simulink model "Copy_of_TenMutantsTemplate"  (R2017b)
settings: Solver=ode3  StartTime=0.0  StopTime=inf  FixedStep=ts  RelTol=0.01  EnableMultiTasking=on
InitFcn:
  | ts=0.0005
  | %ts=100e-6;
StartFcn:
  | close all
StopFcn:
  | % Speed Torque Characterstic
  | 
  | 
  | %figure('Units','pixels', ...
  | %'Color',[1 1 1], ...
  | %'Name','Speed Torque Characterstic',...
  | %'NumberTitle','off',...
  | %'Position',[400 50 470 300], ...
  | %'ToolBar','none');
  | 
  | 
  | 
  | %plot(N_pi,Te_pi)
  | %title('Speed Torque Characterstic')
  | %xlabel('Speed [ RPM ]')
  | %ylabel('Electromagnetic Te_pi [ Nm ] ')
  | %grid on
  | %clear p4 p7 param5 param6 param8 parametres visible voltage
  | 
  | 
  | %clc
values from neighbouring files (symbols this model uses):
  TestOrder = [i]    [ExecuteTestSuite.m]    (also in mutants.m)
undefined symbols (not defined in the file or in its folder): emergency_button2, emergency_buttons, tc_simul, tc_size, temperature, trans1, trans2, trans3, trans4
libraries: simulink x44, powerlib_extras x11
(part 3 of 5)

== system Copy_of_TenMutantsTemplate/mutant7/PI Control1 ==
  N* : Inport
  N : Inport  Port=2
  Abs : Abs  SaturateOnIntegerOverflow=on
  Abs1 : Abs  SaturateOnIntegerOverflow=on
  Abs2 : Abs
  Compare To Constant : simulink/Logic and Bit Operations/Compare To Constant  relop=<=  const=0.1  OutDataTypeStr=uint8
  Constant : Constant  Value=0
  Divide : Product  Inputs=/*
  Integrator Limited : Integrator  LimitOutput=on  UpperSaturationLimit=30  LowerSaturationLimit=-30
  Proportional gain : Gain  Gain=0.8  SaturateOnIntegerOverflow=on  OutDataTypeStr=Inherit: Same as input  ParamDataTypeStr=Inherit: Same as input
  Rate Transition3 : RateTransition  OutPortSampleTimeOpt=Inherit
  Saturation : Saturate  UpperLimit=inf  LowerLimit=2
  Saturation2 : Saturate  UpperLimit=120  LowerLimit=0.02
  Sum1 : Sum  Inputs=|+-  SaturateOnIntegerOverflow=on  InputSameDT=on  OutDataTypeStr=Inherit: Same as first input
  Sum2 : Sum  SaturateOnIntegerOverflow=on  InputSameDT=on  OutDataTypeStr=Inherit: Same as first input
  Sum3 : Sum  Inputs=|++  SaturateOnIntegerOverflow=on  InputSameDT=on  OutDataTypeStr=Inherit: Same as first input
  Switch : Switch  Threshold=0.5
  ctrl_sat : Saturate  UpperLimit=30  LowerLimit=-30
  rpm2hz : Gain  Gain=4/120  SaturateOnIntegerOverflow=on  OutDataTypeStr=Inherit: Same as input  ParamDataTypeStr=Inherit: Same as input
  "rpm2hz  " : Gain  Gain=4/120  SaturateOnIntegerOverflow=on  OutDataTypeStr=Inherit: Same as input  ParamDataTypeStr=Inherit: Same as input
  Freq* : Outport
  wires:
  Saturation/1 -> Divide/1
  Switch/1 -> Integrator Limited/1
  Constant/1 -> Switch/3
  Compare To Constant/1 -> Switch/2
  Abs2/1 -> Divide/2
  Divide/1 -> Compare To Constant/1
  Integrator Limited/1 -> Sum2/1
  N/1 -> "rpm2hz  "/1
  Abs1/1 -> Sum1/2, Sum3/2
  Rate Transition3/1 -> Freq*/1
  Abs/1 -> Sum1/1, Saturation/1
  Sum1/1 -> Abs2/1, Switch/1, Proportional gain/1
  Saturation2/1 -> Rate Transition3/1
  "rpm2hz  "/1 -> Abs1/1
  Proportional gain/1 -> Sum2/2
  rpm2hz/1 -> Abs/1
  ctrl_sat/1 -> Sum3/1
  Sum3/1 -> Saturation2/1
  Sum2/1 -> ctrl_sat/1
  N*/1 -> rpm2hz/1

== system Copy_of_TenMutantsTemplate/mutant7/Subsystem ==
  Speed : Inport
  EmergButton1 : Inport  Port=2
  EmergButton2 : Inport  Port=3
  Temperature : Inport  Port=4
  Compare To Constant : simulink/Logic and Bit Operations/Compare To Constant  relop=>  const=100  OutDataTypeStr=boolean
  Compare To Constant1 : simulink/Logic and Bit Operations/Compare To Constant  relop===  const=0  OutDataTypeStr=boolean
  Constant : Constant  Value=emergency_buttons
  Constant1 : Constant  Value=temperature
  Constant2 : Constant  Value=emergency_button2
  Ir_a3 : Scope
  Logical Operator : Logic  Operator=OR  AllPortsSameDT=off  OutDataTypeStr=boolean
  Logical Operator1 : Logic  AllPortsSameDT=off  OutDataTypeStr=boolean
  Logical Operator2 : Logic  AllPortsSameDT=off  OutDataTypeStr=boolean
  Logical Operator3 : Logic  AllPortsSameDT=off  OutDataTypeStr=boolean
  Speed_to_0 : Constant  Value=0
  Switch : Switch  Criteria=u2 ~= 0
  Switch1 : Switch  Criteria=u2 ~= 0
  Switch2 : Switch  Criteria=u2 ~= 0
  Transfer Fcn1 : TransferFcn  Denominator=[20 1]
  "MotorSpeed " : Outport
  wires:
  EmergButton1/1 -> Logical Operator/1
  EmergButton2/1 -> Logical Operator3/1
  Logical Operator/1 -> Logical Operator1/1
  Speed/1 -> Transfer Fcn1/1
  Switch/1 -> Switch1/3
  Speed_to_0/1 -> Switch1/1, Switch/1
  Logical Operator1/1 -> Switch/2
  Constant/1 -> Logical Operator1/2
  Temperature/1 -> Compare To Constant/1
  Compare To Constant/1 -> Logical Operator2/1
  Constant1/1 -> Logical Operator2/2
  Logical Operator2/1 -> Switch1/2
  Logical Operator3/1 -> Logical Operator/2
  Constant2/1 -> Logical Operator3/2
  Switch1/1 -> Switch2/3, Switch2/1, Compare To Constant1/1
  Switch2/1 -> Ir_a3/1, "MotorSpeed "/1
  Compare To Constant1/1 -> Switch2/2
  Transfer Fcn1/1 -> Switch/3

== system Copy_of_TenMutantsTemplate/mutant7/VSI ==
  Freq : Inport
  Fcn : Fcn  Expr=(2*sqrt(2/3)*Vdc/3)*(2*u(1)-u(2)-u(3))
  Fcn1 : Fcn  Expr=(2*sqrt(2/3)*Vdc/3)*(2*u(2)-u(3)-u(1))
  Fcn2 : Fcn  Expr=(2*sqrt(2/3)*Vdc/3)*(2*u(3)-u(2)-u(1))
  SPWM : Subsystem
  Va : Outport
  Vb : Outport  Port=2
  Vc : Outport  Port=3
  wires:
  SPWM/1(g) -> Fcn2/1, Fcn/1, Fcn1/1
  Fcn1/1 -> Vb/1
  Fcn2/1 -> Vc/1
  Fcn/1 -> Va/1
  Freq/1 -> SPWM/1(Freq)

== system Copy_of_TenMutantsTemplate/mutant8/1 HP , 220 V Induction Motor ==
  tau : Inport
  V_a : Inport  Port=2
  V_b : Inport  Port=3
  V_c : Inport  Port=4
  Flux : Subsystem
  Measurements : Subsystem
  Mechanical : Subsystem
  Mux : Mux  Inputs=3
  Mux1 : Mux  Inputs=3
  abc to dq : Subsystem
  d_block : Subsystem
  dq to abc : Subsystem
  "dq to abc " : Subsystem
  q_block : Subsystem
  rad2rpm : Gain  Gain=30/pi
  m : Outport
  wires:
  Measurements/1(m) -> m/1
  rad2rpm/1 -> Measurements/8(N)
  Mux1/1 -> Measurements/2(I_r)
  Mux/1 -> Measurements/1(I_s)
  "dq to abc "/2(i_rb) -> Mux1/2
  "dq to abc "/3(i_rc) -> Mux1/3
  dq to abc/3(i_sc) -> Mux/3
  dq to abc/2(i_sb) -> Mux/2
  "dq to abc "/1(i_ra) -> Mux1/1
  dq to abc/1(i_sa) -> Mux/1
  V_a/1 -> abc to dq/1(Va)
  V_b/1 -> abc to dq/2(Vb)
  V_c/1 -> abc to dq/3(Vc)
  abc to dq/2(V_qs) -> Flux/2(V_qs)
  abc to dq/1(V_ds) -> Flux/1(V_ds)
  Flux/3(shi_qs) -> Mechanical/2(shi_qs), q_block/1(shi_qs)
  Flux/2("shi_dr ") -> d_block/2(shi_dr)
  tau/1 -> Mechanical/5(tau)
  Mechanical/1(Te) -> Measurements/7(Te)
  q_block/1(i_qs) -> Flux/5(I_qs), dq to abc/2(I_q), Measurements/5(I_qs), Measurements/4(I_dr), Mechanical/4(i_qs)
  q_block/2(i_qr) -> Flux/6(I_qr), "dq to abc "/2(I_q), Measurements/6(I_qr)
  d_block/2(i_dr) -> "dq to abc "/1(I_d), Flux/4(I_dr)
  d_block/1(i_ds) -> Flux/3(I_ds), dq to abc/1(I_d), Measurements/3(I_ds), Mechanical/3(i_ds)
  Flux/4("shi_qr ") -> q_block/2(shi_qr)
  Flux/1(shi_ds) -> Mechanical/1(shi_ds), d_block/1(shi_ds)
  Mechanical/3(we) -> Flux/7(we)
  Mechanical/2(omegaR) -> rad2rpm/1

== system Copy_of_TenMutantsTemplate/mutant8/Data Acquision ==
  note: DONE TO HAVE AN ALLOWABLE SIMULATION TIME
  m : Inport
  speed : Inport  Port=2
  2nd-Order Filter : powerlib_extras/Control  Blocks/2nd-Order Filter  FilterType=Lowpass  Fo=120  Zeta=0.707  Initialize=off  Vac_Init=[1 45 60]  Vdc_Init=-0.5  PlotResponse=off  param1=[1 500 1]
  Bus Selector : BusSelector  OutputSignals=Mechanical.Rotor Speed in (rpm),Mechanical.Electromagnetic Torque (N*m),Stator Measurement.Stator Current i_sa (A)
  Mux : Mux  Inputs=2
  filtroPasaBajos : TransferFcn  Denominator=[1 1]
  is_a : Outport
  Te(Nm) : Outport  Port=2
  wm : Outport  Port=3
  wm1 : Outport  Port=4
  wires:
  filtroPasaBajos/1 -> Mux/1, wm1/1
  Mux/1 -> wm/1
  speed/1 -> Mux/2
  Bus Selector/3 -> is_a/1  "<Stator Current i_sa (A)>"
  Bus Selector/1 -> filtroPasaBajos/1  "<Rotor Speed in (rpm)>"
  m/1 -> Bus Selector/1
  Bus Selector/2 -> 2nd-Order Filter/1  "<Electromagnetic Torque (N*m)>"
  2nd-Order Filter/1 -> Te(Nm)/1

== system Copy_of_TenMutantsTemplate/mutant8/PI Control1 ==
  N* : Inport
  N : Inport  Port=2
  Abs : Abs  SaturateOnIntegerOverflow=on
  Abs1 : Abs  SaturateOnIntegerOverflow=on
  Abs2 : Abs
  Compare To Constant : simulink/Logic and Bit Operations/Compare To Constant  relop=<=  const=0.1  OutDataTypeStr=uint8
  Constant : Constant  Value=0
  Divide : Product  Inputs=/*
  Integrator Limited : Integrator  LimitOutput=on  UpperSaturationLimit=30  LowerSaturationLimit=-30
  Proportional gain : Gain  Gain=0.8  SaturateOnIntegerOverflow=on  OutDataTypeStr=Inherit: Same as input  ParamDataTypeStr=Inherit: Same as input
  Rate Transition3 : RateTransition  OutPortSampleTimeOpt=Inherit
  Saturation : Saturate  UpperLimit=inf  LowerLimit=2
  Saturation2 : Saturate  UpperLimit=120  LowerLimit=0.02
  Sum1 : Sum  Inputs=|+-  SaturateOnIntegerOverflow=on  InputSameDT=on  OutDataTypeStr=Inherit: Same as first input
  Sum2 : Sum  SaturateOnIntegerOverflow=on  InputSameDT=on  OutDataTypeStr=Inherit: Same as first input
  Sum3 : Sum  Inputs=|++  SaturateOnIntegerOverflow=on  InputSameDT=on  OutDataTypeStr=Inherit: Same as first input
  Switch : Switch  Threshold=0.5
  ctrl_sat : Saturate  UpperLimit=30  LowerLimit=-30
  rpm2hz : Gain  Gain=4/120  SaturateOnIntegerOverflow=on  OutDataTypeStr=Inherit: Same as input  ParamDataTypeStr=Inherit: Same as input
  "rpm2hz  " : Gain  Gain=4/120  SaturateOnIntegerOverflow=on  OutDataTypeStr=Inherit: Same as input  ParamDataTypeStr=Inherit: Same as input
  Freq* : Outport
  wires:
  N*/1 -> rpm2hz/1
  Sum2/1 -> ctrl_sat/1
  Sum3/1 -> Saturation2/1
  ctrl_sat/1 -> Sum3/1
  rpm2hz/1 -> Abs/1
  Proportional gain/1 -> Sum2/2
  "rpm2hz  "/1 -> Abs1/1
  Saturation2/1 -> Rate Transition3/1
  Sum1/1 -> Proportional gain/1, Switch/1, Abs2/1
  Abs/1 -> Saturation/1, Sum1/1
  Rate Transition3/1 -> Freq*/1
  Abs1/1 -> Sum3/2, Sum1/2
  N/1 -> "rpm2hz  "/1
  Integrator Limited/1 -> Sum2/1
  Divide/1 -> Compare To Constant/1
  Abs2/1 -> Divide/2
  Compare To Constant/1 -> Switch/2
  Constant/1 -> Switch/3
  Switch/1 -> Integrator Limited/1
  Saturation/1 -> Divide/1

== system Copy_of_TenMutantsTemplate/mutant8/Subsystem ==
  Speed : Inport
  EmergButton1 : Inport  Port=2
  EmergButton2 : Inport  Port=3
  Temperature : Inport  Port=4
  Compare To Constant : simulink/Logic and Bit Operations/Compare To Constant  relop=>  const=100  OutDataTypeStr=boolean
  Compare To Constant1 : simulink/Logic and Bit Operations/Compare To Constant  relop===  const=0  OutDataTypeStr=boolean
  Constant : Constant  Value=emergency_buttons
  Constant1 : Constant  Value=temperature
  Constant2 : Constant  Value=emergency_button2
  Ir_a3 : Scope
  Logical Operator : Logic  Operator=OR  AllPortsSameDT=off  OutDataTypeStr=boolean
  Logical Operator1 : Logic  AllPortsSameDT=off  OutDataTypeStr=boolean
  Logical Operator2 : Logic  AllPortsSameDT=off  OutDataTypeStr=boolean
  Logical Operator3 : Logic  AllPortsSameDT=off  OutDataTypeStr=boolean
  Speed_to_0 : Constant  Value=0
  Switch : Switch  Criteria=u2 ~= 0
  Switch1 : Switch  Criteria=u2 ~= 0
  Switch2 : Switch  Criteria=u2 ~= 0
  Transfer Fcn1 : TransferFcn  Denominator=[20 1]
  "MotorSpeed " : Outport
  wires:
  Transfer Fcn1/1 -> Switch/3
  Compare To Constant1/1 -> Switch2/2
  Switch2/1 -> "MotorSpeed "/1, Ir_a3/1
  Switch1/1 -> Compare To Constant1/1, Switch2/1, Switch2/3
  Constant2/1 -> Logical Operator3/2
  Logical Operator3/1 -> Logical Operator/2
  Logical Operator2/1 -> Switch1/2
  Constant1/1 -> Logical Operator2/2
  Compare To Constant/1 -> Logical Operator2/1
  Temperature/1 -> Compare To Constant/1
  Constant/1 -> Logical Operator1/2
  Logical Operator1/1 -> Switch/2
  Speed_to_0/1 -> Switch/1, Switch1/1
  Switch/1 -> Switch1/3
  Speed/1 -> Transfer Fcn1/1
  Logical Operator/1 -> Logical Operator1/1
  EmergButton2/1 -> Logical Operator3/1
  EmergButton1/1 -> Logical Operator/1

== system Copy_of_TenMutantsTemplate/mutant8/VSI ==
  Freq : Inport
  Fcn : Fcn  Expr=(2*sqrt(2/3)*Vdc/3)*(2*u(1)-u(2)-u(3))
  Fcn1 : Fcn  Expr=(2*sqrt(2/3)*Vdc/3)*(2*u(2)-u(3)-u(1))
  Fcn2 : Fcn  Expr=(2*sqrt(2/3)*Vdc/3)*(2*u(3)-u(2)-u(1))
  SPWM : Subsystem
  Va : Outport
  Vb : Outport  Port=2
  Vc : Outport  Port=3
  wires:
  Freq/1 -> SPWM/1(Freq)
  Fcn/1 -> Va/1
  Fcn2/1 -> Vc/1
  Fcn1/1 -> Vb/1
  SPWM/1(g) -> Fcn1/1, Fcn/1, Fcn2/1

== system Copy_of_TenMutantsTemplate/mutant9/1 HP , 220 V Induction Motor ==
  tau : Inport
  V_a : Inport  Port=2
  V_b : Inport  Port=3
  V_c : Inport  Port=4
  Flux : Subsystem
  Measurements : Subsystem
  Mechanical : Subsystem
  Mux : Mux  Inputs=3
  Mux1 : Mux  Inputs=3
  abc to dq : Subsystem
  d_block : Subsystem
  dq to abc : Subsystem
  "dq to abc " : Subsystem
  q_block : Subsystem
  rad2rpm : Gain  Gain=30/pi
  m : Outport
  wires:
  Mechanical/2(omegaR) -> rad2rpm/1
  Mechanical/3(we) -> Flux/7(we)
  Flux/1(shi_ds) -> d_block/1(shi_ds), Mechanical/1(shi_ds)
  Flux/4("shi_qr ") -> q_block/2(shi_qr)
  d_block/1(i_ds) -> Mechanical/3(i_ds), Measurements/3(I_ds), dq to abc/1(I_d), Flux/3(I_ds)
  d_block/2(i_dr) -> Flux/4(I_dr), "dq to abc "/1(I_d)
  q_block/2(i_qr) -> Measurements/6(I_qr), "dq to abc "/2(I_q), Flux/6(I_qr)
  q_block/1(i_qs) -> Mechanical/4(i_qs), Measurements/4(I_dr), Measurements/5(I_qs), dq to abc/2(I_q), Flux/5(I_qs)
  Mechanical/1(Te) -> Measurements/7(Te)
  tau/1 -> Mechanical/5(tau)
  Flux/2("shi_dr ") -> d_block/2(shi_dr)
  Flux/3(shi_qs) -> q_block/1(shi_qs), Mechanical/2(shi_qs)
  abc to dq/1(V_ds) -> Flux/1(V_ds)
  abc to dq/2(V_qs) -> Flux/2(V_qs)
  V_c/1 -> abc to dq/3(Vc)
  V_b/1 -> abc to dq/2(Vb)
  V_a/1 -> abc to dq/1(Va)
  dq to abc/1(i_sa) -> Mux/1
  "dq to abc "/1(i_ra) -> Mux1/1
  dq to abc/2(i_sb) -> Mux/2
  dq to abc/3(i_sc) -> Mux/3
  "dq to abc "/3(i_rc) -> Mux1/3
  "dq to abc "/2(i_rb) -> Mux1/2
  Mux/1 -> Measurements/1(I_s)
  Mux1/1 -> Measurements/2(I_r)
  rad2rpm/1 -> Measurements/8(N)
  Measurements/1(m) -> m/1

== system Copy_of_TenMutantsTemplate/mutant9/Data Acquision ==
  note: DONE TO HAVE AN ALLOWABLE SIMULATION TIME
  m : Inport
  speed : Inport  Port=2
  2nd-Order Filter : powerlib_extras/Control  Blocks/2nd-Order Filter  FilterType=Lowpass  Fo=120  Zeta=0.707  Initialize=off  Vac_Init=[1 45 60]  Vdc_Init=-0.5  PlotResponse=off  param1=[1 500 1]
  Bus Selector : BusSelector  OutputSignals=Mechanical.Rotor Speed in (rpm),Mechanical.Electromagnetic Torque (N*m),Stator Measurement.Stator Current i_sa (A)
  Mux : Mux  Inputs=2
  filtroPasaBajos : TransferFcn  Denominator=[1 1]
  is_a : Outport
  Te(Nm) : Outport  Port=2
  wm : Outport  Port=3
  wm1 : Outport  Port=4
  wires:
  2nd-Order Filter/1 -> Te(Nm)/1
  Bus Selector/2 -> 2nd-Order Filter/1  "<Electromagnetic Torque (N*m)>"
  m/1 -> Bus Selector/1
  Bus Selector/1 -> filtroPasaBajos/1  "<Rotor Speed in (rpm)>"
  Bus Selector/3 -> is_a/1  "<Stator Current i_sa (A)>"
  speed/1 -> Mux/2
  Mux/1 -> wm/1
  filtroPasaBajos/1 -> wm1/1, Mux/1

== system Copy_of_TenMutantsTemplate/mutant9/PI Control1 ==
  N* : Inport
  N : Inport  Port=2
  Abs : Abs  SaturateOnIntegerOverflow=on
  Abs1 : Abs  SaturateOnIntegerOverflow=on
  Abs2 : Abs
  Compare To Constant : simulink/Logic and Bit Operations/Compare To Constant  relop=<=  const=0.1  OutDataTypeStr=uint8
  Constant : Constant  Value=0
  Divide : Product  Inputs=/*
  Integrator Limited : Integrator  LimitOutput=on  UpperSaturationLimit=30  LowerSaturationLimit=-30
  Proportional gain : Gain  Gain=0.8  SaturateOnIntegerOverflow=on  OutDataTypeStr=Inherit: Same as input  ParamDataTypeStr=Inherit: Same as input
  Rate Transition3 : RateTransition  OutPortSampleTimeOpt=Inherit
  Saturation : Saturate  UpperLimit=inf  LowerLimit=2
  Saturation2 : Saturate  UpperLimit=120  LowerLimit=0.02
  Sum1 : Sum  Inputs=|+-  SaturateOnIntegerOverflow=on  InputSameDT=on  OutDataTypeStr=Inherit: Same as first input
  Sum2 : Sum  SaturateOnIntegerOverflow=on  InputSameDT=on  OutDataTypeStr=Inherit: Same as first input
  Sum3 : Sum  Inputs=|++  SaturateOnIntegerOverflow=on  InputSameDT=on  OutDataTypeStr=Inherit: Same as first input
  Switch : Switch  Threshold=0.5
  ctrl_sat : Saturate  UpperLimit=30  LowerLimit=-30
  rpm2hz : Gain  Gain=4/120  SaturateOnIntegerOverflow=on  OutDataTypeStr=Inherit: Same as input  ParamDataTypeStr=Inherit: Same as input
  "rpm2hz  " : Gain  Gain=4/120  SaturateOnIntegerOverflow=on  OutDataTypeStr=Inherit: Same as input  ParamDataTypeStr=Inherit: Same as input
  Freq* : Outport
  wires:
  Saturation/1 -> Divide/1
  Switch/1 -> Integrator Limited/1
  Constant/1 -> Switch/3
  Compare To Constant/1 -> Switch/2
  Abs2/1 -> Divide/2
  Divide/1 -> Compare To Constant/1
  Integrator Limited/1 -> Sum2/1
  N/1 -> "rpm2hz  "/1
  Abs1/1 -> Sum1/2, Sum3/2
  Rate Transition3/1 -> Freq*/1
  Abs/1 -> Sum1/1, Saturation/1
  Sum1/1 -> Abs2/1, Switch/1, Proportional gain/1
  Saturation2/1 -> Rate Transition3/1
  "rpm2hz  "/1 -> Abs1/1
  Proportional gain/1 -> Sum2/2
  rpm2hz/1 -> Abs/1
  ctrl_sat/1 -> Sum3/1
  Sum3/1 -> Saturation2/1
  Sum2/1 -> ctrl_sat/1
  N*/1 -> rpm2hz/1

== system Copy_of_TenMutantsTemplate/mutant9/Subsystem ==
  Speed : Inport
  EmergButton1 : Inport  Port=2
  EmergButton2 : Inport  Port=3
  Temperature : Inport  Port=4
  Compare To Constant : simulink/Logic and Bit Operations/Compare To Constant  relop=>  const=100  OutDataTypeStr=boolean
  Compare To Constant1 : simulink/Logic and Bit Operations/Compare To Constant  relop===  const=0  OutDataTypeStr=boolean
  Constant : Constant  Value=emergency_buttons
  Constant1 : Constant  Value=temperature
  Constant2 : Constant  Value=emergency_button2
  Ir_a3 : Scope
  Logical Operator : Logic  Operator=OR  AllPortsSameDT=off  OutDataTypeStr=boolean
  Logical Operator1 : Logic  AllPortsSameDT=off  OutDataTypeStr=boolean
  Logical Operator2 : Logic  AllPortsSameDT=off  OutDataTypeStr=boolean
  Logical Operator3 : Logic  AllPortsSameDT=off  OutDataTypeStr=boolean
  Speed_to_0 : Constant  Value=0
  Switch : Switch  Criteria=u2 ~= 0
  Switch1 : Switch  Criteria=u2 ~= 0
  Switch2 : Switch  Criteria=u2 ~= 0
  Transfer Fcn1 : TransferFcn  Denominator=[20 1]
  "MotorSpeed " : Outport
  wires:
  EmergButton1/1 -> Logical Operator/1
  EmergButton2/1 -> Logical Operator3/1
  Logical Operator/1 -> Logical Operator1/1
  Speed/1 -> Transfer Fcn1/1
  Switch/1 -> Switch1/3
  Speed_to_0/1 -> Switch1/1, Switch/1
  Logical Operator1/1 -> Switch/2
  Constant/1 -> Logical Operator1/2
  Temperature/1 -> Compare To Constant/1
  Compare To Constant/1 -> Logical Operator2/1
  Constant1/1 -> Logical Operator2/2
  Logical Operator2/1 -> Switch1/2
  Logical Operator3/1 -> Logical Operator/2
  Constant2/1 -> Logical Operator3/2
  Switch1/1 -> Switch2/3, Switch2/1, Compare To Constant1/1
  Switch2/1 -> Ir_a3/1, "MotorSpeed "/1
  Compare To Constant1/1 -> Switch2/2
  Transfer Fcn1/1 -> Switch/3

== system Copy_of_TenMutantsTemplate/mutant9/VSI ==
  Freq : Inport
  Fcn : Fcn  Expr=(2*sqrt(2/3)*Vdc/3)*(2*u(1)-u(2)-u(3))
  Fcn1 : Fcn  Expr=(2*sqrt(2/3)*Vdc/3)*(2*u(2)-u(3)-u(1))
  Fcn2 : Fcn  Expr=(2*sqrt(2/3)*Vdc/3)*(2*u(3)-u(2)-u(1))
  SPWM : Subsystem
  Va : Outport
  Vb : Outport  Port=2
  Vc : Outport  Port=3
  wires:
  SPWM/1(g) -> Fcn2/1, Fcn/1, Fcn1/1
  Fcn1/1 -> Vb/1
  Fcn2/1 -> Vc/1
  Fcn/1 -> Va/1
  Freq/1 -> SPWM/1(Freq)

== system Copy_of_TenMutantsTemplate/System/1 HP , 220 V Induction Motor/Flux ==
  V_ds : Inport
  V_qs : Inport  Port=2
  I_ds : Inport  Port=3
  I_dr : Inport  Port=4
  I_qs : Inport  Port=5
  I_qr : Inport  Port=6
  we : Inport  Port=7
  Integrator{,1..3} (4 alike) : Integrator
  Product : Product
  Product1 : Product
  Rr : Gain  Gain=Rr
  "Rr " : Gain  Gain=Rr
  Rs : Gain  Gain=Rs
  "Rs " : Gain  Gain=Rs
  Sum : Sum  Inputs=+|-
  Sum1 : Sum  Inputs=+|-
  Sum2 : Sum  Inputs=|--
  Sum3 : Sum  Inputs=|+-
  shi_ds : Outport
  "shi_dr " : Outport  Port=2
  shi_qs : Outport  Port=3
  "shi_qr " : Outport  Port=4
  wires:
  Sum3/1 -> Integrator3/1
  "Rr "/1 -> Sum3/2
  Product1/1 -> Sum3/1
  I_qr/1 -> "Rr "/1
  Integrator2/1 -> "shi_dr "/1, Product1/2
  Sum2/1 -> Integrator2/1
  Product/1 -> Sum2/1
  Rr/1 -> Sum2/2
  I_dr/1 -> Rr/1
  Integrator3/1 -> "shi_qr "/1, Product/1
  we/1 -> Product1/1, Product/2
  "Rs "/1 -> Sum1/2
  Rs/1 -> Sum/2
  Integrator1/1 -> shi_qs/1
  Integrator/1 -> shi_ds/1
  Sum1/1 -> Integrator1/1
  V_qs/1 -> Sum1/1
  I_qs/1 -> "Rs "/1
  Sum/1 -> Integrator/1
  V_ds/1 -> Sum/1
  I_ds/1 -> Rs/1

== system Copy_of_TenMutantsTemplate/System/1 HP , 220 V Induction Motor/Measurements ==
  I_s : Inport
  I_r : Inport  Port=2
  I_ds : Inport  Port=3
  I_dr : Inport  Port=4
  I_qs : Inport  Port=5
  I_qr : Inport  Port=6
  Te : Inport  Port=7
  N : Inport  Port=8
  Bus Creator : BusCreator  Inputs=5
  Bus Creator1 : BusCreator  Inputs=5
  Bus Creator2 : BusCreator  Inputs=2
  Bus Creator3 : BusCreator  Inputs=3
  Demux : Demux  Outputs=3
  Demux1 : Demux  Outputs=3
  m : Outport
  wires:
  Bus Creator3/1 -> m/1
  Bus Creator2/1 -> Bus Creator3/3  "Mechanical"
  Bus Creator1/1 -> Bus Creator3/2  "Rotor Measurement"
  Bus Creator/1 -> Bus Creator3/1  "Stator Measurement"
  N/1 -> Bus Creator2/2  "Rotor Speed in (rpm)"
  Te/1 -> Bus Creator2/1  "Electromagnetic Torque (N*m)"
  I_qr/1 -> Bus Creator1/5  "Rotor Current i_qs (A)"
  I_dr/1 -> Bus Creator1/4  "Rotor Current i_ds (A)"
  Demux1/3 -> Bus Creator1/3  "Rotor Current i_sc (A)"
  Demux1/2 -> Bus Creator1/2  "Rotor Current i_sb (A)"
  Demux1/1 -> Bus Creator1/1  "Rotor Current i_sa (A)"
  I_r/1 -> Demux1/1
  I_qs/1 -> Bus Creator/5  "Stator Current i_qs (A)"
  I_ds/1 -> Bus Creator/4  "Stator Current i_ds (A)"
  Demux/3 -> Bus Creator/3  "Stator Current i_sc (A)"
  Demux/2 -> Bus Creator/2  "Stator Current i_sb (A)"
  Demux/1 -> Bus Creator/1  "Stator Current i_sa (A)"
  I_s/1 -> Demux/1

== system Copy_of_TenMutantsTemplate/System/1 HP , 220 V Induction Motor/Mechanical ==
  shi_ds : Inport
  shi_qs : Inport  Port=2
  i_ds : Inport  Port=3
  i_qs : Inport  Port=4
  tau : Inport  Port=5
  " " : Gain  Gain=P/2  SaturateOnIntegerOverflow=on  OutDataTypeStr=Inherit: Same as input  ParamDataTypeStr=Inherit: Same as input
  "  " : Gain  Gain=3*P/4  SaturateOnIntegerOverflow=on  OutDataTypeStr=Inherit: Same as input  ParamDataTypeStr=Inherit: Same as input
  1/J : Gain  Gain=1/J  SaturateOnIntegerOverflow=on  OutDataTypeStr=Inherit: Same as input  ParamDataTypeStr=Inherit: Same as input
  Integratorw : Integrator
  Product1 : Product
  Product2 : Product
  Sum : Sum  Inputs=+|-
  Sum5 : Sum  Inputs=+-  SaturateOnIntegerOverflow=on  InputSameDT=on  OutDataTypeStr=Inherit: Same as first input
  Te : Outport
  omegaR : Outport  Port=2
  we : Outport  Port=3
  wires:
  " "/1 -> we/1
  Integratorw/1 -> omegaR/1, " "/1
  1/J/1 -> Integratorw/1
  Sum5/1 -> 1/J/1
  tau/1 -> Sum5/2
  "  "/1 -> Sum5/1, Te/1
  Sum/1 -> "  "/1
  Product2/1 -> Sum/1
  Product1/1 -> Sum/2
  i_ds/1 -> Product1/2
  shi_qs/1 -> Product1/1
  i_qs/1 -> Product2/2
  shi_ds/1 -> Product2/1

== system Copy_of_TenMutantsTemplate/System/1 HP , 220 V Induction Motor/abc to dq ==
  Va : Inport
  Vb : Inport  Port=2
  Vc : Inport  Port=3
  "            " : Terminator
  Demux : Demux  Outputs=3
  Mux : Mux  Inputs=3
  abc2dq : Gain  Gain=[2/3 -1/3 -1/3; 0 sqrt(3)/3 -sqrt(3)/3; 1/3 1/3 1/3]  Multiplication=Matrix(K*u)  SaturateOnIntegerOverflow=on  OutDataTypeStr=Inherit: Same as input  ParamDataTypeStr=Inherit: Same as input
  V_ds : Outport
  V_qs : Outport  Port=2
  wires:
  Mux/1 -> abc2dq/1
  abc2dq/1 -> Demux/1
  Demux/2 -> V_qs/1
  Demux/1 -> V_ds/1
  Va/1 -> Mux/1
  Vb/1 -> Mux/2
  Vc/1 -> Mux/3
  Demux/3 -> "            "/1

== system Copy_of_TenMutantsTemplate/System/1 HP , 220 V Induction Motor/d_block ==
  shi_ds : Inport
  shi_dr : Inport  Port=2
  1/(Lr-((Lm*Lm)/Ls)) : Gain  Gain=1/(Lr-((Lm*Lm)/Ls))  SaturateOnIntegerOverflow=on  OutDataTypeStr=Inherit: Same as input  ParamDataTypeStr=Inherit: Same as input
  1/(Ls-((Lm*Lm)/Lr)) : Gain  Gain=1/(Ls-((Lm*Lm)/Lr))  SaturateOnIntegerOverflow=on  OutDataTypeStr=Inherit: Same as input  ParamDataTypeStr=Inherit: Same as input
  Lm/Lr : Gain  Gain=Lm/Lr
  Lm/Ls : Gain  Gain=Lm/Ls
  Sum : Sum  Inputs=|+-
  Sum1 : Sum  Inputs=-+|
  i_ds : Outport
  i_dr : Outport  Port=2
  wires:
  Sum1/1 -> 1/(Lr-((Lm*Lm)/Ls))/1
  Lm/Ls/1 -> Sum1/1
  Sum/1 -> 1/(Ls-((Lm*Lm)/Lr))/1
  Lm/Lr/1 -> Sum/2
  shi_dr/1 -> Sum1/2, Lm/Lr/1
  shi_ds/1 -> Lm/Ls/1, Sum/1
  1/(Lr-((Lm*Lm)/Ls))/1 -> i_dr/1
  1/(Ls-((Lm*Lm)/Lr))/1 -> i_ds/1

== system Copy_of_TenMutantsTemplate/System/1 HP , 220 V Induction Motor/dq to abc ==
  I_d : Inport
  I_q : Inport  Port=2
  Demux : Demux  Outputs=3
  Gain : Gain  Gain=2/3  SaturateOnIntegerOverflow=on  OutDataTypeStr=Inherit: Same as input  ParamDataTypeStr=Inherit: Same as input
  Matrix Gain : Gain  Gain=[1 0;-0.5 -sqrt(3)/2;-0.5 sqrt(3)/2]  Multiplication=Matrix(K*u)  SaturateOnIntegerOverflow=on  OutDataTypeStr=Inherit: Same as input  ParamDataTypeStr=Inherit: Same as input
  Mux : Mux  Inputs=2
  i_sa : Outport
  i_sb : Outport  Port=2
  i_sc : Outport  Port=3
  wires:
  Demux/1 -> i_sa/1
  Demux/3 -> i_sc/1
  I_q/1 -> Mux/2
  I_d/1 -> Mux/1
  Demux/2 -> i_sb/1
  Matrix Gain/1 -> Gain/1
  Gain/1 -> Demux/1
  Mux/1 -> Matrix Gain/1

== system Copy_of_TenMutantsTemplate/System/1 HP , 220 V Induction Motor/dq to abc  ==
  I_d : Inport
  I_q : Inport  Port=2
  Demux : Demux  Outputs=3
  Gain : Gain  Gain=2/3  SaturateOnIntegerOverflow=on  OutDataTypeStr=Inherit: Same as input  ParamDataTypeStr=Inherit: Same as input
  Matrix Gain : Gain  Gain=[1 0;-0.5 -sqrt(3)/2;-0.5 sqrt(3)/2]  Multiplication=Matrix(K*u)  SaturateOnIntegerOverflow=on  OutDataTypeStr=Inherit: Same as input  ParamDataTypeStr=Inherit: Same as input
  Mux : Mux  Inputs=2
  i_ra : Outport
  i_rb : Outport  Port=2
  i_rc : Outport  Port=3
  wires:
  Mux/1 -> Matrix Gain/1
  Gain/1 -> Demux/1
  Matrix Gain/1 -> Gain/1
  Demux/2 -> i_rb/1
  I_d/1 -> Mux/1
  I_q/1 -> Mux/2
  Demux/3 -> i_rc/1
  Demux/1 -> i_ra/1

== system Copy_of_TenMutantsTemplate/System/1 HP , 220 V Induction Motor/q_block ==
  shi_qs : Inport
  shi_qr : Inport  Port=2
  1/(Lr-((Lm*Lm)/Ls)) : Gain  Gain=1/(Lr-((Lm*Lm)/Ls))  SaturateOnIntegerOverflow=on  OutDataTypeStr=Inherit: Same as input  ParamDataTypeStr=Inherit: Same as input
  1/(Ls-((Lm*Lm)/Lr)) : Gain  Gain=1/(Ls-((Lm*Lm)/Lr))  SaturateOnIntegerOverflow=on  OutDataTypeStr=Inherit: Same as input  ParamDataTypeStr=Inherit: Same as input
  Lm/Lr : Gain  Gain=Lm/Lr
  Lm/Ls : Gain  Gain=Lm/Ls
  Sum : Sum  Inputs=|+-
  Sum1 : Sum  Inputs=-+|
  i_qs : Outport
  i_qr : Outport  Port=2
  wires:
  Sum1/1 -> 1/(Lr-((Lm*Lm)/Ls))/1
  Lm/Ls/1 -> Sum1/1
  Sum/1 -> 1/(Ls-((Lm*Lm)/Lr))/1
  Lm/Lr/1 -> Sum/2
  shi_qr/1 -> Lm/Lr/1, Sum1/2
  shi_qs/1 -> Lm/Ls/1, Sum/1
  1/(Lr-((Lm*Lm)/Ls))/1 -> i_qr/1
  1/(Ls-((Lm*Lm)/Lr))/1 -> i_qs/1

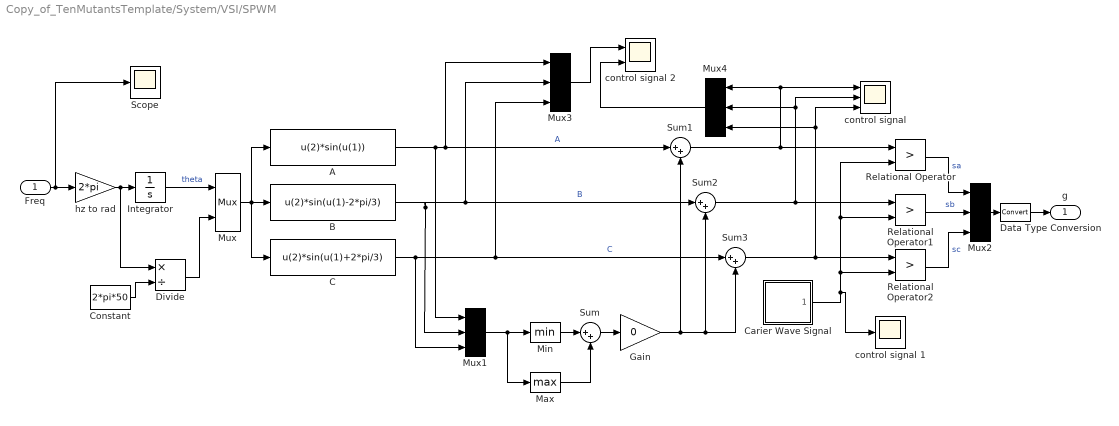
== system Copy_of_TenMutantsTemplate/System/VSI/SPWM ==
  Freq : Inport
  A : Fcn  Expr=u(2)*sin(u(1))
  B : Fcn  Expr=u(2)*sin(u(1)-2*pi/3)
  C : Fcn  Expr=u(2)*sin(u(1)+2*pi/3)
  Carier Wave Signal : Subsystem  mask(Carrier Wave Generator:){A=1, fc=500}
      mask prompts: A "Amplitude"; fc "Carrier Wave Frequency"
      mask Display: fprintf('Carrier\nWave')
  Constant : Constant  Value=2*pi*50
  Data Type Conversion : DataTypeConversion
  Divide : Product  Inputs=*/
  Gain : Gain  Gain=0
  Integrator : Integrator
  Max : MinMax  Function=max
  Min : MinMax
  Mux : Mux  Inputs=2
      settings: DisplayOption=signals
  Mux{1..4} (4 alike) : Mux  Inputs=3
      settings: DisplayOption=signals
  Relational Operator : RelationalOperator  Operator=>  OutDataTypeStr=boolean  RndMeth=Nearest
  Relational Operator1 : RelationalOperator  Operator=>  OutDataTypeStr=boolean  RndMeth=Nearest
  Relational Operator2 : RelationalOperator  Operator=>  OutDataTypeStr=boolean  RndMeth=Nearest
  Scope : Scope
  Sum{,1..3} (4 alike) : Sum  Inputs=|++
  "control signal " : Scope  NumInputPorts=3
  control signal 1 : Scope
  control signal 2 : Scope  NumInputPorts=2
  hz to rad : Gain  Gain=2*pi
  g : Outport
  wires:
  Mux4/1 -> control signal 2/2
  Mux3/1 -> control signal 2/1
  Constant/1 -> Divide/2
  Divide/1 -> Mux/2
  Gain/1 -> Sum1/2, Sum3/2, Sum2/2
  Freq/1 -> hz to rad/1, Scope/1
  C/1 -> Mux3/3, Sum3/1, Mux1/3  "C"
  Mux/1 -> C/1, A/1, B/1
  Integrator/1 -> Mux/1  "theta"
  A/1 -> Mux3/1, Sum1/1, Mux1/1  "A"
  hz to rad/1 -> Divide/1, Integrator/1
  B/1 -> Mux3/2, Sum2/1, Mux1/2  "B"
  Min/1 -> Sum/1
  Max/1 -> Sum/2
  Carier Wave Signal/1("Carier Wave ") -> control signal 1/1, Relational Operator2/2, Relational Operator1/2, Relational Operator/2
  Relational Operator2/1 -> Mux2/3  "sc"
  Relational Operator1/1 -> Mux2/2  "sb"
  Relational Operator/1 -> Mux2/1  "sa"
  Mux1/1 -> Max/1, Min/1
  Sum/1 -> Gain/1
  Sum1/1 -> Mux4/1, "control signal "/1, Relational Operator/1
  Sum2/1 -> Mux4/2, "control signal "/2, Relational Operator1/1
  Sum3/1 -> Mux4/3, "control signal "/3, Relational Operator2/1
  Mux2/1 -> Data Type Conversion/1
  Data Type Conversion/1 -> g/1

== system Copy_of_TenMutantsTemplate/mutant1/1 HP , 220 V Induction Motor/Flux ==
  V_ds : Inport
  V_qs : Inport  Port=2
  I_ds : Inport  Port=3
  I_dr : Inport  Port=4
  I_qs : Inport  Port=5
  I_qr : Inport  Port=6
  we : Inport  Port=7
  Integrator{,1..3} (4 alike) : Integrator
  Product : Product
  Product1 : Product
  Rr : Gain  Gain=Rr
  "Rr " : Gain  Gain=Rr
  Rs : Gain  Gain=Rs
  "Rs " : Gain  Gain=Rs
  Sum : Sum  Inputs=+|-
  Sum1 : Sum  Inputs=+|-
  Sum2 : Sum  Inputs=|--
  Sum3 : Sum  Inputs=|+-
  shi_ds : Outport
  "shi_dr " : Outport  Port=2
  shi_qs : Outport  Port=3
  "shi_qr " : Outport  Port=4
  wires:
  I_ds/1 -> Rs/1
  V_ds/1 -> Sum/1
  Sum/1 -> Integrator/1
  I_qs/1 -> "Rs "/1
  V_qs/1 -> Sum1/1
  Sum1/1 -> Integrator1/1
  Integrator/1 -> shi_ds/1
  Integrator1/1 -> shi_qs/1
  Rs/1 -> Sum/2
  "Rs "/1 -> Sum1/2
  we/1 -> Product/2, Product1/1
  Integrator3/1 -> Product/1, "shi_qr "/1
  I_dr/1 -> Rr/1
  Rr/1 -> Sum2/2
  Product/1 -> Sum2/1
  Sum2/1 -> Integrator2/1
  Integrator2/1 -> Product1/2, "shi_dr "/1
  I_qr/1 -> "Rr "/1
  Product1/1 -> Sum3/1
  "Rr "/1 -> Sum3/2
  Sum3/1 -> Integrator3/1

== system Copy_of_TenMutantsTemplate/mutant1/1 HP , 220 V Induction Motor/Measurements ==
  I_s : Inport
  I_r : Inport  Port=2
  I_ds : Inport  Port=3
  I_dr : Inport  Port=4
  I_qs : Inport  Port=5
  I_qr : Inport  Port=6
  Te : Inport  Port=7
  N : Inport  Port=8
  Bus Creator : BusCreator  Inputs=5
  Bus Creator1 : BusCreator  Inputs=5
  Bus Creator2 : BusCreator  Inputs=2
  Bus Creator3 : BusCreator  Inputs=3
  Demux : Demux  Outputs=3
  Demux1 : Demux  Outputs=3
  m : Outport
  wires:
  I_s/1 -> Demux/1
  Demux/1 -> Bus Creator/1  "Stator Current i_sa (A)"
  Demux/2 -> Bus Creator/2  "Stator Current i_sb (A)"
  Demux/3 -> Bus Creator/3  "Stator Current i_sc (A)"
  I_ds/1 -> Bus Creator/4  "Stator Current i_ds (A)"
  I_qs/1 -> Bus Creator/5  "Stator Current i_qs (A)"
  I_r/1 -> Demux1/1
  Demux1/1 -> Bus Creator1/1  "Rotor Current i_sa (A)"
  Demux1/2 -> Bus Creator1/2  "Rotor Current i_sb (A)"
  Demux1/3 -> Bus Creator1/3  "Rotor Current i_sc (A)"
  I_dr/1 -> Bus Creator1/4  "Rotor Current i_ds (A)"
  I_qr/1 -> Bus Creator1/5  "Rotor Current i_qs (A)"
  Te/1 -> Bus Creator2/1  "Electromagnetic Torque (N*m)"
  N/1 -> Bus Creator2/2  "Rotor Speed in (rpm)"
  Bus Creator/1 -> Bus Creator3/1  "Stator Measurement"
  Bus Creator1/1 -> Bus Creator3/2  "Rotor Measurement"
  Bus Creator2/1 -> Bus Creator3/3  "Mechanical"
  Bus Creator3/1 -> m/1

== system Copy_of_TenMutantsTemplate/mutant1/1 HP , 220 V Induction Motor/Mechanical ==
  shi_ds : Inport
  shi_qs : Inport  Port=2
  i_ds : Inport  Port=3
  i_qs : Inport  Port=4
  tau : Inport  Port=5
  " " : Gain  Gain=P/2  SaturateOnIntegerOverflow=on  OutDataTypeStr=Inherit: Same as input  ParamDataTypeStr=Inherit: Same as input
  "  " : Gain  Gain=3*P/4  SaturateOnIntegerOverflow=on  OutDataTypeStr=Inherit: Same as input  ParamDataTypeStr=Inherit: Same as input
  1/J : Gain  Gain=1/J  SaturateOnIntegerOverflow=on  OutDataTypeStr=Inherit: Same as input  ParamDataTypeStr=Inherit: Same as input
  Integratorw : Integrator
  Product1 : Product
  Product2 : Product
  Sum : Sum  Inputs=+|-
  Sum5 : Sum  Inputs=+-  SaturateOnIntegerOverflow=on  InputSameDT=on  OutDataTypeStr=Inherit: Same as first input
  Te : Outport
  omegaR : Outport  Port=2
  we : Outport  Port=3
  wires:
  shi_ds/1 -> Product2/1
  i_qs/1 -> Product2/2
  shi_qs/1 -> Product1/1
  i_ds/1 -> Product1/2
  Product1/1 -> Sum/2
  Product2/1 -> Sum/1
  Sum/1 -> "  "/1
  "  "/1 -> Te/1, Sum5/1
  tau/1 -> Sum5/2
  Sum5/1 -> 1/J/1
  1/J/1 -> Integratorw/1
  Integratorw/1 -> " "/1, omegaR/1
  " "/1 -> we/1

== system Copy_of_TenMutantsTemplate/mutant1/1 HP , 220 V Induction Motor/abc to dq ==
  Va : Inport
  Vb : Inport  Port=2
  Vc : Inport  Port=3
  "            " : Terminator
  Demux : Demux  Outputs=3
  Mux : Mux  Inputs=3
  abc2dq : Gain  Gain=[2/3 -1/3 -1/3; 0 sqrt(3)/3 -sqrt(3)/3; 1/3 1/3 1/3]  Multiplication=Matrix(K*u)  SaturateOnIntegerOverflow=on  OutDataTypeStr=Inherit: Same as input  ParamDataTypeStr=Inherit: Same as input
  V_ds : Outport
  V_qs : Outport  Port=2
  wires:
  Demux/3 -> "            "/1
  Vc/1 -> Mux/3
  Vb/1 -> Mux/2
  Va/1 -> Mux/1
  Demux/1 -> V_ds/1
  Demux/2 -> V_qs/1
  abc2dq/1 -> Demux/1
  Mux/1 -> abc2dq/1

== system Copy_of_TenMutantsTemplate/mutant1/1 HP , 220 V Induction Motor/d_block ==
  shi_ds : Inport
  shi_dr : Inport  Port=2
  1/(Lr-((Lm*Lm)/Ls)) : Gain  Gain=1/(Lr-((Lm*Lm)/Ls))  SaturateOnIntegerOverflow=on  OutDataTypeStr=Inherit: Same as input  ParamDataTypeStr=Inherit: Same as input
  1/(Ls-((Lm*Lm)/Lr)) : Gain  Gain=1/(Ls-((Lm*Lm)/Lr))  SaturateOnIntegerOverflow=on  OutDataTypeStr=Inherit: Same as input  ParamDataTypeStr=Inherit: Same as input
  Lm/Lr : Gain  Gain=Lm/Lr
  Lm/Ls : Gain  Gain=Lm/Ls
  Sum : Sum  Inputs=|+-
  Sum1 : Sum  Inputs=-+|
  i_ds : Outport
  i_dr : Outport  Port=2
  wires:
  1/(Ls-((Lm*Lm)/Lr))/1 -> i_ds/1
  1/(Lr-((Lm*Lm)/Ls))/1 -> i_dr/1
  shi_ds/1 -> Sum/1, Lm/Ls/1
  shi_dr/1 -> Lm/Lr/1, Sum1/2
  Lm/Lr/1 -> Sum/2
  Sum/1 -> 1/(Ls-((Lm*Lm)/Lr))/1
  Lm/Ls/1 -> Sum1/1
  Sum1/1 -> 1/(Lr-((Lm*Lm)/Ls))/1

== system Copy_of_TenMutantsTemplate/mutant1/1 HP , 220 V Induction Motor/dq to abc ==
  I_d : Inport
  I_q : Inport  Port=2
  Demux : Demux  Outputs=3
  Gain : Gain  Gain=2/3  SaturateOnIntegerOverflow=on  OutDataTypeStr=Inherit: Same as input  ParamDataTypeStr=Inherit: Same as input
  Matrix Gain : Gain  Gain=[1 0;-0.5 -sqrt(3)/2;-0.5 sqrt(3)/2]  Multiplication=Matrix(K*u)  SaturateOnIntegerOverflow=on  OutDataTypeStr=Inherit: Same as input  ParamDataTypeStr=Inherit: Same as input
  Mux : Mux  Inputs=2
  i_sa : Outport
  i_sb : Outport  Port=2
  i_sc : Outport  Port=3
  wires:
  Mux/1 -> Matrix Gain/1
  Gain/1 -> Demux/1
  Matrix Gain/1 -> Gain/1
  Demux/2 -> i_sb/1
  I_d/1 -> Mux/1
  I_q/1 -> Mux/2
  Demux/3 -> i_sc/1
  Demux/1 -> i_sa/1

== system Copy_of_TenMutantsTemplate/mutant1/1 HP , 220 V Induction Motor/dq to abc  ==
  I_d : Inport
  I_q : Inport  Port=2
  Demux : Demux  Outputs=3
  Gain : Gain  Gain=2/3  SaturateOnIntegerOverflow=on  OutDataTypeStr=Inherit: Same as input  ParamDataTypeStr=Inherit: Same as input
  Matrix Gain : Gain  Gain=[1 0;-0.5 -sqrt(3)/2;-0.5 sqrt(3)/2]  Multiplication=Matrix(K*u)  SaturateOnIntegerOverflow=on  OutDataTypeStr=Inherit: Same as input  ParamDataTypeStr=Inherit: Same as input
  Mux : Mux  Inputs=2
  i_ra : Outport
  i_rb : Outport  Port=2
  i_rc : Outport  Port=3
  wires:
  Demux/1 -> i_ra/1
  Demux/3 -> i_rc/1
  I_q/1 -> Mux/2
  I_d/1 -> Mux/1
  Demux/2 -> i_rb/1
  Matrix Gain/1 -> Gain/1
  Gain/1 -> Demux/1
  Mux/1 -> Matrix Gain/1

== system Copy_of_TenMutantsTemplate/mutant1/1 HP , 220 V Induction Motor/q_block ==
  shi_qs : Inport
  shi_qr : Inport  Port=2
  1/(Lr-((Lm*Lm)/Ls)) : Gain  Gain=1/(Lr-((Lm*Lm)/Ls))  SaturateOnIntegerOverflow=on  OutDataTypeStr=Inherit: Same as input  ParamDataTypeStr=Inherit: Same as input
  1/(Ls-((Lm*Lm)/Lr)) : Gain  Gain=1/(Ls-((Lm*Lm)/Lr))  SaturateOnIntegerOverflow=on  OutDataTypeStr=Inherit: Same as input  ParamDataTypeStr=Inherit: Same as input
  Lm/Lr : Gain  Gain=Lm/Lr
  Lm/Ls : Gain  Gain=Lm/Ls
  Sum : Sum  Inputs=|+-
  Sum1 : Sum  Inputs=-+|
  i_qs : Outport
  i_qr : Outport  Port=2
  wires:
  1/(Ls-((Lm*Lm)/Lr))/1 -> i_qs/1
  1/(Lr-((Lm*Lm)/Ls))/1 -> i_qr/1
  shi_qs/1 -> Sum/1, Lm/Ls/1
  shi_qr/1 -> Sum1/2, Lm/Lr/1
  Lm/Lr/1 -> Sum/2
  Sum/1 -> 1/(Ls-((Lm*Lm)/Lr))/1
  Lm/Ls/1 -> Sum1/1
  Sum1/1 -> 1/(Lr-((Lm*Lm)/Ls))/1

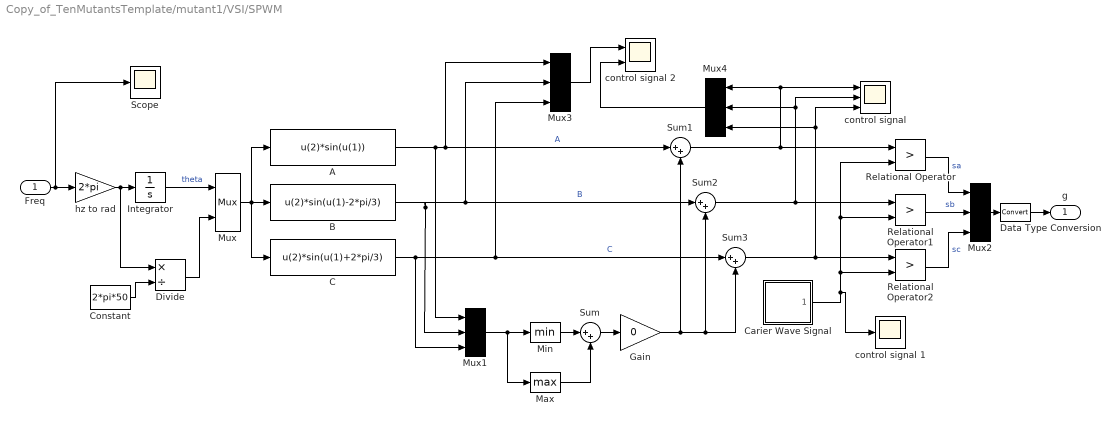
== system Copy_of_TenMutantsTemplate/mutant1/VSI/SPWM ==
  Freq : Inport
  A : Fcn  Expr=u(2)*sin(u(1))
  B : Fcn  Expr=u(2)*sin(u(1)-2*pi/3)
  C : Fcn  Expr=u(2)*sin(u(1)+2*pi/3)
  Carier Wave Signal : Subsystem  mask(Carrier Wave Generator:){A=1, fc=500}
      mask prompts: A "Amplitude"; fc "Carrier Wave Frequency"
      mask Display: fprintf('Carrier\nWave')
  Constant : Constant  Value=2*pi*50
  Data Type Conversion : DataTypeConversion
  Divide : Product  Inputs=*/
  Gain : Gain  Gain=0
  Integrator : Integrator
  Max : MinMax  Function=max
  Min : MinMax
  Mux : Mux  Inputs=2
      settings: DisplayOption=signals
  Mux{1..4} (4 alike) : Mux  Inputs=3
      settings: DisplayOption=signals
  Relational Operator : RelationalOperator  Operator=>  OutDataTypeStr=boolean  RndMeth=Nearest
  Relational Operator1 : RelationalOperator  Operator=>  OutDataTypeStr=boolean  RndMeth=Nearest
  Relational Operator2 : RelationalOperator  Operator=>  OutDataTypeStr=boolean  RndMeth=Nearest
  Scope : Scope
  Sum{,1..3} (4 alike) : Sum  Inputs=|++
  "control signal " : Scope  NumInputPorts=3
  control signal 1 : Scope
  control signal 2 : Scope  NumInputPorts=2
  hz to rad : Gain  Gain=2*pi
  g : Outport
  wires:
  Data Type Conversion/1 -> g/1
  Mux2/1 -> Data Type Conversion/1
  Sum3/1 -> Relational Operator2/1, "control signal "/3, Mux4/3
  Sum2/1 -> Relational Operator1/1, "control signal "/2, Mux4/2
  Sum1/1 -> Relational Operator/1, "control signal "/1, Mux4/1
  Sum/1 -> Gain/1
  Mux1/1 -> Min/1, Max/1
  Relational Operator/1 -> Mux2/1  "sa"
  Relational Operator1/1 -> Mux2/2  "sb"
  Relational Operator2/1 -> Mux2/3  "sc"
  Carier Wave Signal/1("Carier Wave ") -> Relational Operator/2, Relational Operator1/2, Relational Operator2/2, control signal 1/1
  Max/1 -> Sum/2
  Min/1 -> Sum/1
  B/1 -> Mux1/2, Sum2/1, Mux3/2  "B"
  hz to rad/1 -> Integrator/1, Divide/1
  A/1 -> Mux1/1, Sum1/1, Mux3/1  "A"
  Integrator/1 -> Mux/1  "theta"
  Mux/1 -> B/1, A/1, C/1
  C/1 -> Mux1/3, Sum3/1, Mux3/3  "C"
  Freq/1 -> Scope/1, hz to rad/1
  Gain/1 -> Sum2/2, Sum3/2, Sum1/2
  Divide/1 -> Mux/2
  Constant/1 -> Divide/2
  Mux3/1 -> control signal 2/1
  Mux4/1 -> control signal 2/2

== system Copy_of_TenMutantsTemplate/mutant10/1 HP , 220 V Induction Motor/Flux ==
  V_ds : Inport
  V_qs : Inport  Port=2
  I_ds : Inport  Port=3
  I_dr : Inport  Port=4
  I_qs : Inport  Port=5
  I_qr : Inport  Port=6
  we : Inport  Port=7
  Integrator{,1..3} (4 alike) : Integrator
  Product : Product
  Product1 : Product
  Rr : Gain  Gain=Rr
  "Rr " : Gain  Gain=Rr
  Rs : Gain  Gain=Rs
  "Rs " : Gain  Gain=Rs
  Sum : Sum  Inputs=+|-
  Sum1 : Sum  Inputs=+|-
  Sum2 : Sum  Inputs=|--
  Sum3 : Sum  Inputs=|+-
  shi_ds : Outport
  "shi_dr " : Outport  Port=2
  shi_qs : Outport  Port=3
  "shi_qr " : Outport  Port=4
  wires:
  I_ds/1 -> Rs/1
  V_ds/1 -> Sum/1
  Sum/1 -> Integrator/1
  I_qs/1 -> "Rs "/1
  V_qs/1 -> Sum1/1
  Sum1/1 -> Integrator1/1
  Integrator/1 -> shi_ds/1
  Integrator1/1 -> shi_qs/1
  Rs/1 -> Sum/2
  "Rs "/1 -> Sum1/2
  we/1 -> Product/2, Product1/1
  Integrator3/1 -> Product/1, "shi_qr "/1
  I_dr/1 -> Rr/1
  Rr/1 -> Sum2/2
  Product/1 -> Sum2/1
  Sum2/1 -> Integrator2/1
  Integrator2/1 -> Product1/2, "shi_dr "/1
  I_qr/1 -> "Rr "/1
  Product1/1 -> Sum3/1
  "Rr "/1 -> Sum3/2
  Sum3/1 -> Integrator3/1

== system Copy_of_TenMutantsTemplate/mutant10/1 HP , 220 V Induction Motor/Measurements ==
  I_s : Inport
  I_r : Inport  Port=2
  I_ds : Inport  Port=3
  I_dr : Inport  Port=4
  I_qs : Inport  Port=5
  I_qr : Inport  Port=6
  Te : Inport  Port=7
  N : Inport  Port=8
  Bus Creator : BusCreator  Inputs=5
  Bus Creator1 : BusCreator  Inputs=5
  Bus Creator2 : BusCreator  Inputs=2
  Bus Creator3 : BusCreator  Inputs=3
  Demux : Demux  Outputs=3
  Demux1 : Demux  Outputs=3
  m : Outport
  wires:
  I_s/1 -> Demux/1
  Demux/1 -> Bus Creator/1  "Stator Current i_sa (A)"
  Demux/2 -> Bus Creator/2  "Stator Current i_sb (A)"
  Demux/3 -> Bus Creator/3  "Stator Current i_sc (A)"
  I_ds/1 -> Bus Creator/4  "Stator Current i_ds (A)"
  I_qs/1 -> Bus Creator/5  "Stator Current i_qs (A)"
  I_r/1 -> Demux1/1
  Demux1/1 -> Bus Creator1/1  "Rotor Current i_sa (A)"
  Demux1/2 -> Bus Creator1/2  "Rotor Current i_sb (A)"
  Demux1/3 -> Bus Creator1/3  "Rotor Current i_sc (A)"
  I_dr/1 -> Bus Creator1/4  "Rotor Current i_ds (A)"
  I_qr/1 -> Bus Creator1/5  "Rotor Current i_qs (A)"
  Te/1 -> Bus Creator2/1  "Electromagnetic Torque (N*m)"
  N/1 -> Bus Creator2/2  "Rotor Speed in (rpm)"
  Bus Creator/1 -> Bus Creator3/1  "Stator Measurement"
  Bus Creator1/1 -> Bus Creator3/2  "Rotor Measurement"
  Bus Creator2/1 -> Bus Creator3/3  "Mechanical"
  Bus Creator3/1 -> m/1

== system Copy_of_TenMutantsTemplate/mutant10/1 HP , 220 V Induction Motor/Mechanical ==
  shi_ds : Inport
  shi_qs : Inport  Port=2
  i_ds : Inport  Port=3
  i_qs : Inport  Port=4
  tau : Inport  Port=5
  " " : Gain  Gain=P/2  SaturateOnIntegerOverflow=on  OutDataTypeStr=Inherit: Same as input  ParamDataTypeStr=Inherit: Same as input
  "  " : Gain  Gain=3*P/4  SaturateOnIntegerOverflow=on  OutDataTypeStr=Inherit: Same as input  ParamDataTypeStr=Inherit: Same as input
  1/J : Gain  Gain=1/J  SaturateOnIntegerOverflow=on  OutDataTypeStr=Inherit: Same as input  ParamDataTypeStr=Inherit: Same as input
  Integratorw : Integrator
  Product1 : Product
  Product2 : Product
  Sum : Sum  Inputs=+|-
  Sum5 : Sum  Inputs=+-  SaturateOnIntegerOverflow=on  InputSameDT=on  OutDataTypeStr=Inherit: Same as first input
  Te : Outport
  omegaR : Outport  Port=2
  we : Outport  Port=3
  wires:
  shi_ds/1 -> Product2/1
  i_qs/1 -> Product2/2
  shi_qs/1 -> Product1/1
  i_ds/1 -> Product1/2
  Product1/1 -> Sum/2
  Product2/1 -> Sum/1
  Sum/1 -> "  "/1
  "  "/1 -> Te/1, Sum5/1
  tau/1 -> Sum5/2
  Sum5/1 -> 1/J/1
  1/J/1 -> Integratorw/1
  Integratorw/1 -> " "/1, omegaR/1
  " "/1 -> we/1

== system Copy_of_TenMutantsTemplate/mutant10/1 HP , 220 V Induction Motor/abc to dq ==
  Va : Inport
  Vb : Inport  Port=2
  Vc : Inport  Port=3
  "            " : Terminator
  Demux : Demux  Outputs=3
  Mux : Mux  Inputs=3
  abc2dq : Gain  Gain=[2/3 -1/3 -1/3; 0 sqrt(3)/3 -sqrt(3)/3; 1/3 1/3 1/3]  Multiplication=Matrix(K*u)  SaturateOnIntegerOverflow=on  OutDataTypeStr=Inherit: Same as input  ParamDataTypeStr=Inherit: Same as input
  V_ds : Outport
  V_qs : Outport  Port=2
  wires:
  Demux/3 -> "            "/1
  Vc/1 -> Mux/3
  Vb/1 -> Mux/2
  Va/1 -> Mux/1
  Demux/1 -> V_ds/1
  Demux/2 -> V_qs/1
  abc2dq/1 -> Demux/1
  Mux/1 -> abc2dq/1

== system Copy_of_TenMutantsTemplate/mutant10/1 HP , 220 V Induction Motor/d_block ==
  shi_ds : Inport
  shi_dr : Inport  Port=2
  1/(Lr-((Lm*Lm)/Ls)) : Gain  Gain=1/(Lr-((Lm*Lm)/Ls))  SaturateOnIntegerOverflow=on  OutDataTypeStr=Inherit: Same as input  ParamDataTypeStr=Inherit: Same as input
  1/(Ls-((Lm*Lm)/Lr)) : Gain  Gain=1/(Ls-((Lm*Lm)/Lr))  SaturateOnIntegerOverflow=on  OutDataTypeStr=Inherit: Same as input  ParamDataTypeStr=Inherit: Same as input
  Lm/Lr : Gain  Gain=Lm/Lr
  Lm/Ls : Gain  Gain=Lm/Ls
  Sum : Sum  Inputs=|+-
  Sum1 : Sum  Inputs=-+|
  i_ds : Outport
  i_dr : Outport  Port=2
  wires:
  1/(Ls-((Lm*Lm)/Lr))/1 -> i_ds/1
  1/(Lr-((Lm*Lm)/Ls))/1 -> i_dr/1
  shi_ds/1 -> Sum/1, Lm/Ls/1
  shi_dr/1 -> Lm/Lr/1, Sum1/2
  Lm/Lr/1 -> Sum/2
  Sum/1 -> 1/(Ls-((Lm*Lm)/Lr))/1
  Lm/Ls/1 -> Sum1/1
  Sum1/1 -> 1/(Lr-((Lm*Lm)/Ls))/1

== system Copy_of_TenMutantsTemplate/mutant10/1 HP , 220 V Induction Motor/dq to abc ==
  I_d : Inport
  I_q : Inport  Port=2
  Demux : Demux  Outputs=3
  Gain : Gain  Gain=2/3  SaturateOnIntegerOverflow=on  OutDataTypeStr=Inherit: Same as input  ParamDataTypeStr=Inherit: Same as input
  Matrix Gain : Gain  Gain=[1 0;-0.5 -sqrt(3)/2;-0.5 sqrt(3)/2]  Multiplication=Matrix(K*u)  SaturateOnIntegerOverflow=on  OutDataTypeStr=Inherit: Same as input  ParamDataTypeStr=Inherit: Same as input
  Mux : Mux  Inputs=2
  i_sa : Outport
  i_sb : Outport  Port=2
  i_sc : Outport  Port=3
  wires:
  Mux/1 -> Matrix Gain/1
  Gain/1 -> Demux/1
  Matrix Gain/1 -> Gain/1
  Demux/2 -> i_sb/1
  I_d/1 -> Mux/1
  I_q/1 -> Mux/2
  Demux/3 -> i_sc/1
  Demux/1 -> i_sa/1

== system Copy_of_TenMutantsTemplate/mutant10/1 HP , 220 V Induction Motor/dq to abc  ==
  I_d : Inport
  I_q : Inport  Port=2
  Demux : Demux  Outputs=3
  Gain : Gain  Gain=2/3  SaturateOnIntegerOverflow=on  OutDataTypeStr=Inherit: Same as input  ParamDataTypeStr=Inherit: Same as input
  Matrix Gain : Gain  Gain=[1 0;-0.5 -sqrt(3)/2;-0.5 sqrt(3)/2]  Multiplication=Matrix(K*u)  SaturateOnIntegerOverflow=on  OutDataTypeStr=Inherit: Same as input  ParamDataTypeStr=Inherit: Same as input
  Mux : Mux  Inputs=2
  i_ra : Outport
  i_rb : Outport  Port=2
  i_rc : Outport  Port=3
  wires:
  Demux/1 -> i_ra/1
  Demux/3 -> i_rc/1
  I_q/1 -> Mux/2
  I_d/1 -> Mux/1
  Demux/2 -> i_rb/1
  Matrix Gain/1 -> Gain/1
  Gain/1 -> Demux/1
  Mux/1 -> Matrix Gain/1

== system Copy_of_TenMutantsTemplate/mutant10/1 HP , 220 V Induction Motor/q_block ==
  shi_qs : Inport
  shi_qr : Inport  Port=2
  1/(Lr-((Lm*Lm)/Ls)) : Gain  Gain=1/(Lr-((Lm*Lm)/Ls))  SaturateOnIntegerOverflow=on  OutDataTypeStr=Inherit: Same as input  ParamDataTypeStr=Inherit: Same as input
  1/(Ls-((Lm*Lm)/Lr)) : Gain  Gain=1/(Ls-((Lm*Lm)/Lr))  SaturateOnIntegerOverflow=on  OutDataTypeStr=Inherit: Same as input  ParamDataTypeStr=Inherit: Same as input
  Lm/Lr : Gain  Gain=Lm/Lr
  Lm/Ls : Gain  Gain=Lm/Ls
  Sum : Sum  Inputs=|+-
  Sum1 : Sum  Inputs=-+|
  i_qs : Outport
  i_qr : Outport  Port=2
  wires:
  1/(Ls-((Lm*Lm)/Lr))/1 -> i_qs/1
  1/(Lr-((Lm*Lm)/Ls))/1 -> i_qr/1
  shi_qs/1 -> Sum/1, Lm/Ls/1
  shi_qr/1 -> Sum1/2, Lm/Lr/1
  Lm/Lr/1 -> Sum/2
  Sum/1 -> 1/(Ls-((Lm*Lm)/Lr))/1
  Lm/Ls/1 -> Sum1/1
  Sum1/1 -> 1/(Lr-((Lm*Lm)/Ls))/1

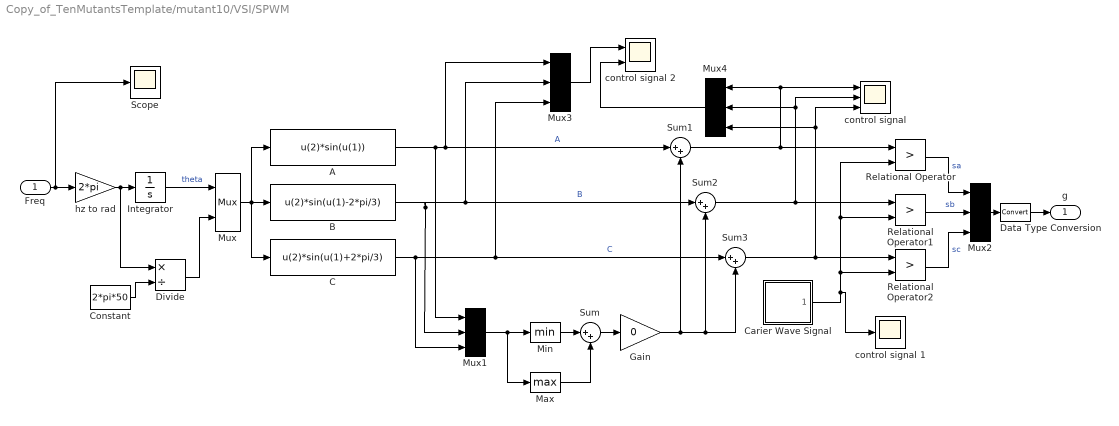
== system Copy_of_TenMutantsTemplate/mutant10/VSI/SPWM ==
  Freq : Inport
  A : Fcn  Expr=u(2)*sin(u(1))
  B : Fcn  Expr=u(2)*sin(u(1)-2*pi/3)
  C : Fcn  Expr=u(2)*sin(u(1)+2*pi/3)
  Carier Wave Signal : Subsystem  mask(Carrier Wave Generator:){A=1, fc=500}
      mask prompts: A "Amplitude"; fc "Carrier Wave Frequency"
      mask Display: fprintf('Carrier\nWave')
  Constant : Constant  Value=2*pi*50
  Data Type Conversion : DataTypeConversion
  Divide : Product  Inputs=*/
  Gain : Gain  Gain=0
  Integrator : Integrator
  Max : MinMax  Function=max
  Min : MinMax
  Mux : Mux  Inputs=2
      settings: DisplayOption=signals
  Mux{1..4} (4 alike) : Mux  Inputs=3
      settings: DisplayOption=signals
  Relational Operator : RelationalOperator  Operator=>  OutDataTypeStr=boolean  RndMeth=Nearest
  Relational Operator1 : RelationalOperator  Operator=>  OutDataTypeStr=boolean  RndMeth=Nearest
  Relational Operator2 : RelationalOperator  Operator=>  OutDataTypeStr=boolean  RndMeth=Nearest
  Scope : Scope
  Sum{,1..3} (4 alike) : Sum  Inputs=|++
  "control signal " : Scope  NumInputPorts=3
  control signal 1 : Scope
  control signal 2 : Scope  NumInputPorts=2
  hz to rad : Gain  Gain=2*pi
  g : Outport
  wires:
  Data Type Conversion/1 -> g/1
  Mux2/1 -> Data Type Conversion/1
  Sum3/1 -> Relational Operator2/1, "control signal "/3, Mux4/3
  Sum2/1 -> Relational Operator1/1, "control signal "/2, Mux4/2
  Sum1/1 -> Relational Operator/1, "control signal "/1, Mux4/1
  Sum/1 -> Gain/1
  Mux1/1 -> Min/1, Max/1
  Relational Operator/1 -> Mux2/1  "sa"
  Relational Operator1/1 -> Mux2/2  "sb"
  Relational Operator2/1 -> Mux2/3  "sc"
  Carier Wave Signal/1("Carier Wave ") -> Relational Operator/2, Relational Operator1/2, Relational Operator2/2, control signal 1/1
  Max/1 -> Sum/2
  Min/1 -> Sum/1
  B/1 -> Mux1/2, Sum2/1, Mux3/2  "B"
  hz to rad/1 -> Integrator/1, Divide/1
  A/1 -> Mux1/1, Sum1/1, Mux3/1  "A"
  Integrator/1 -> Mux/1  "theta"
  Mux/1 -> B/1, A/1, C/1
  C/1 -> Mux1/3, Sum3/1, Mux3/3  "C"
  Freq/1 -> Scope/1, hz to rad/1
  Gain/1 -> Sum2/2, Sum3/2, Sum1/2
  Divide/1 -> Mux/2
  Constant/1 -> Divide/2
  Mux3/1 -> control signal 2/1
  Mux4/1 -> control signal 2/2

== system Copy_of_TenMutantsTemplate/mutant2/1 HP , 220 V Induction Motor/Flux ==
  V_ds : Inport
  V_qs : Inport  Port=2
  I_ds : Inport  Port=3
  I_dr : Inport  Port=4
  I_qs : Inport  Port=5
  I_qr : Inport  Port=6
  we : Inport  Port=7
  Integrator{,1..3} (4 alike) : Integrator
  Product : Product
  Product1 : Product
  Rr : Gain  Gain=Rr
  "Rr " : Gain  Gain=Rr
  Rs : Gain  Gain=Rs
  "Rs " : Gain  Gain=Rs
  Sum : Sum  Inputs=+|-
  Sum1 : Sum  Inputs=+|-
  Sum2 : Sum  Inputs=|--
  Sum3 : Sum  Inputs=|+-
  shi_ds : Outport
  "shi_dr " : Outport  Port=2
  shi_qs : Outport  Port=3
  "shi_qr " : Outport  Port=4
  wires:
  Sum3/1 -> Integrator3/1
  "Rr "/1 -> Sum3/2
  Product1/1 -> Sum3/1
  I_qr/1 -> "Rr "/1
  Integrator2/1 -> "shi_dr "/1, Product1/2
  Sum2/1 -> Integrator2/1
  Product/1 -> Sum2/1
  Rr/1 -> Sum2/2
  I_dr/1 -> Rr/1
  Integrator3/1 -> "shi_qr "/1, Product/1
  we/1 -> Product1/1, Product/2
  "Rs "/1 -> Sum1/2
  Rs/1 -> Sum/2
  Integrator1/1 -> shi_qs/1
  Integrator/1 -> shi_ds/1
  Sum1/1 -> Integrator1/1
  V_qs/1 -> Sum1/1
  I_qs/1 -> "Rs "/1
  Sum/1 -> Integrator/1
  V_ds/1 -> Sum/1
  I_ds/1 -> Rs/1
